simulink model "lab2_simulink"  (R2021b)
settings: Solver=VariableStepAuto  StartTime=0.0  StopTime=10.0  RelTol=1e-3
undefined symbols (not defined in the file): K, licz, mian
settings Model: Creator=szczy  LastModifiedBy=szczy

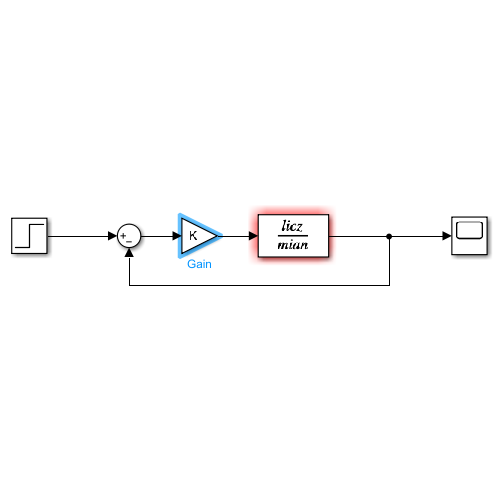
[thumbnail: Simulink's stored preview of the top-level diagram]
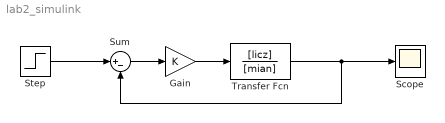
== system lab2_simulink ==
  Gain : Gain  Gain=K
  Scope : Scope
  Step : Step  SampleTime=0
  Sum : Sum  Inputs=|+-
  Transfer Fcn : TransferFcn  Numerator=[licz]  Denominator=[mian]
  wires:
  Sum/1 -> Gain/1
  Gain/1 -> Transfer Fcn/1
  Transfer Fcn/1 -> Sum/2, Scope/1
  Step/1 -> Sum/1
